simulink model "VTOL_sim"  (R2016b)
settings: Solver=ode45  StartTime=0.0  StopTime=200  RelTol=1e-3  EnableMultiTasking=on
InitFcn:
  | addpath ./..
  | VTOL_param
  | VTOLParamHW10
undefined symbols (not defined in the file or in its folder): P, VTOL_animation, VTOL_ctrl
settings Model: Creator=beard  LastModifiedBy=beard
settings DataIOCC: LimitDataPoints=on  SaveFormat=Array  SignalLoggingSaveFormat=ModelDataLogs
settings OptimizationCC: ExpressionDepthLimit=2147483647  InitFltsAndDblsToZero=on  LifeSpan=inf
settings DebuggingCC: UnderspecifiedInitializationDetection=Classic  MergeDetectMultiDrivingBlocksExec=none  SolverPrmCheckMsg=warning  FcnCallInpInsideContextMsg=warning  StateNameClashWarn=warning  SFUnexpectedBacktrackingDiag=warning  SFNoUnconditionalDefaultTransitionDiag=warning  SFExecutionAtInitializationDiag=none
settings HardwareCC: ProdBitPerPointer=32  ProdBitPerSizeT=32  ProdBitPerPtrDiffT=32  ProdLargestAtomicFloat=None  ProdIntDivRoundTo=Undefined  ProdEndianess=Unspecified  ProdWordSize=32  ProdHWDeviceType=32-bit Generic
settings ModelReferenceCC: PropagateSignalLabelsOutOfModel=off
settings GRTTargetCC: TargetLangStandard=C89/C90 (ANSI)  GeneratePreprocessorConditionals=Disable all  CombineOutputUpdateFcns=off  GRTInterface=on
settings ConfigComp: CovMetricSettings=dw  CovHtmlReporting=on  CovSaveCumulativeToWorkspaceVar=on  CovSaveSingleToWorkspaceVar=on  CovExternalEMLEnable=off

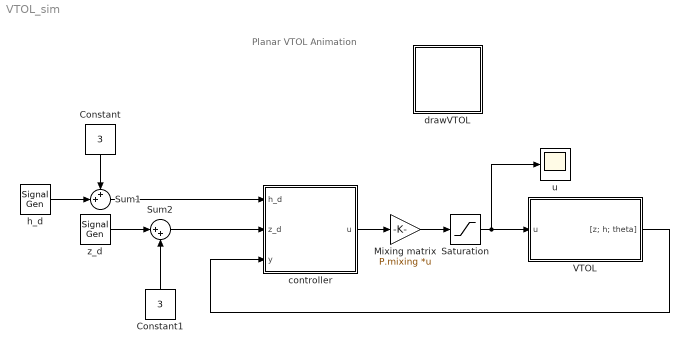
== system VTOL_sim ==
  note: Planar VTOL Animation
  Constant : Constant  Value=3
  Constant1 : Constant  Value=3
  Mixing matrix : Gain  Gain=P.mixing  Multiplication=Matrix(K*u)
  Saturation : Saturate  UpperLimit=P.fmax  LowerLimit=0
  Sum1 : Sum  Inputs=++|
  Sum2 : Sum  Inputs=|++
  VTOL : Subsystem
  controller : Subsystem
  drawVTOL : Subsystem
      mask Display: image(imread('tv.jpg'))
  h_d : SignalGenerator  WaveForm=square  Amplitude=2.5  Frequency=.02
  u : Scope
  z_d : SignalGenerator  WaveForm=square  Amplitude=2.5  Frequency=.008
  wires:
  VTOL/1("[z; h; theta]") -> controller/3(y)
  Constant/1 -> Sum1/1
  h_d/1 -> Sum1/2
  Sum2/1 -> controller/2(z_d)
  z_d/1 -> Sum2/1
  Constant1/1 -> Sum2/2
  Saturation/1 -> VTOL/1(u), u/1
  Mixing matrix/1 -> Saturation/1
  controller/1(u) -> Mixing matrix/1
  Sum1/1 -> controller/1(h_d)

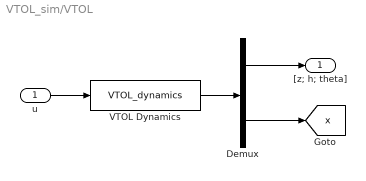
== system VTOL_sim/VTOL ==
  u : Inport
  Demux : Demux  Outputs=[3;6]
  VTOL Dynamics : S-Function  FunctionName=VTOL_dynamics  Parameters=P  SFunctionDeploymentMode=off  EnableBusSupport=off
  "[z; h; theta]" : Outport
  tag scope: x=global
  wires:
  Demux/2 -> [x]
  Demux/1 -> "[z; h; theta]"/1
  VTOL Dynamics/1 -> Demux/1
  u/1 -> VTOL Dynamics/1

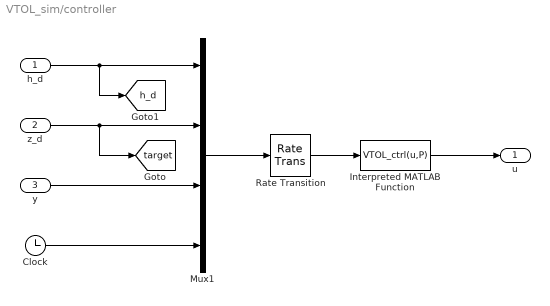
== system VTOL_sim/controller ==
  h_d : Inport
  z_d : Inport  Port=2
  y : Inport  Port=3
  Clock : Clock
  Interpreted MATLAB Function : MATLABFcn  MATLABFcn=VTOL_ctrl(u,P)  OutputDimensions=2
  Mux1 : Mux
  Rate Transition : RateTransition  OutPortSampleTime=P.Ts
  u : Outport
  tag scope: h_d=global, target=global
  wires:
  Mux1/1 -> Rate Transition/1
  h_d/1 -> [h_d], Mux1/1
  Interpreted MATLAB Function/1 -> u/1
  Clock/1 -> Mux1/4
  Rate Transition/1 -> Interpreted MATLAB Function/1
  y/1 -> Mux1/3
  z_d/1 -> [target], Mux1/2

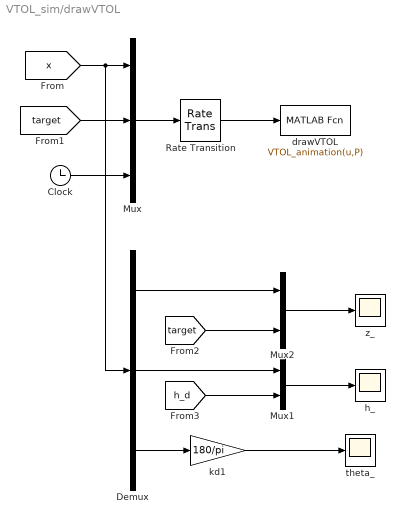
== system VTOL_sim/drawVTOL ==
  Clock : Clock
  Demux : Demux  Outputs=3
  Mux : Mux  Inputs=3
  Mux1 : Mux  Inputs=2
  Mux2 : Mux  Inputs=2
  Rate Transition : RateTransition  OutPortSampleTime=P.t_plot
  drawVTOL : MATLABFcn  MATLABFcn=VTOL_animation(u,P)  OutputDimensions=0
  h_ : Scope
  kd1 : Gain  Gain=180/pi
  theta_ : Scope
  z_ : Scope
  wires:
  [target] -> Mux/2
  Rate Transition/1 -> drawVTOL/1
  Clock/1 -> Mux/3
  Mux/1 -> Rate Transition/1
  [x] -> Demux/1, Mux/1
  Mux1/1 -> h_/1
  Mux2/1 -> z_/1
  kd1/1 -> theta_/1
  Demux/3 -> kd1/1
  Demux/1 -> Mux2/1
  [target] -> Mux2/2
  Demux/2 -> Mux1/1
  [h_d] -> Mux1/2
